simulink model "lab12"  (R2022b)
settings: Solver=VariableStepAuto  StartTime=0.0  StopTime=100  RelTol=1e-3
values from neighbouring files (symbols this model uses):
  m = 5    [lab3_1.m]    (also in lab43_2.m = 200)
  n = 7    [lab3_1.m]    (also in test.m = length(polynomial1_bin); test_OCMC.m = length(seq1))
libraries: simulink x2, dspstat3 x1
settings Model: Creator=user  LastModifiedBy=user

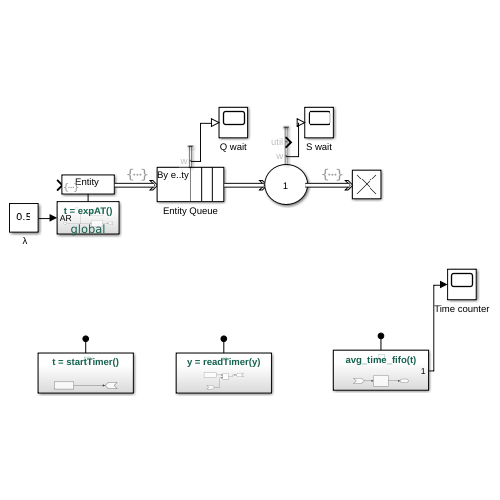
[thumbnail: Simulink's stored preview of the top-level diagram]
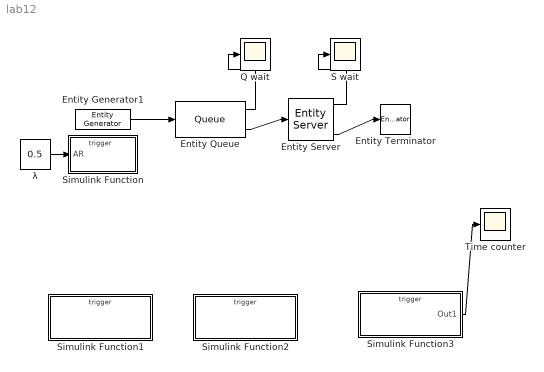
== system lab12 ==
  " λ" : Constant  Value=0.5  SampleTime=-1
  Entity Generator1 : EntityGenerator  OutputPortMessageModes=m  TimeSource=Signal port  IntergenerationTimeAction=dt = expAT();  GenerateAction=|  AttributeName=ServiceTime|Timer  AttributeInitialValue=0|0  EntityType=Structured  EntityTypeName=Entity
      | entity.ServiceTime = exprnd(3);
      | entitySys.priority = randi(2);
      | entity.Timer = 0; % Инициализация Timer
      | entity.Timer = startTimer(); % Запуск таймера
      settings: InputPortMap=u1
  Entity Queue : Queue  InputPortMessageModes=m  OutputPortMessageModes=n,m  Capacity=100  QueueType=Priority  PrioritySource=entitySys.priority  EntryAction=entity.Timer = startTimer();  AverageWait=on
      settings: OutputPortMap=o2,o5
  Entity Server : EntityServer  InputPortMessageModes=m  OutputPortMessageModes=n,n,m  Capacity=1  ServiceTimeSource=Attribute  AverageWait=on  Utilization=on
      settings: OutputPortMap=o4,o5,o9
  Entity Terminator : EntityTerminator  InputPortMessageModes=m  EntryAction=|
      | elapsedTime = readTimer(entity.Timer);
      | avg_time_fifo(elapsedTime);
  Q wait : Scope
  S wait : Scope
  Simulink Function : Subsystem  TreatAsAtomicUnit=on
      settings: LibrarySourceBlock=sldelib/Simulink Function
  Simulink Function1 : Subsystem  TreatAsAtomicUnit=on
  Simulink Function2 : Subsystem  TreatAsAtomicUnit=on
  Simulink Function3 : Subsystem  TreatAsAtomicUnit=on
  Time counter : Scope
  wires:
  " λ"/1 -> Simulink Function/1(AR)
  Entity Generator1/1 -> Entity Queue/1
  Entity Queue/2 -> Entity Server/1
  Entity Server/3 -> Entity Terminator/1
  Simulink Function3/1(Out1) -> Time counter/1
  Entity Server/1 -> S wait/1
  Entity Queue/1 -> Q wait/1

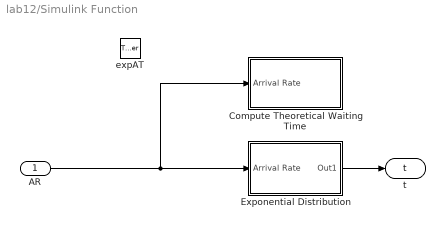
== system lab12/Simulink Function ==
  AR : Inport
  expAT : TriggerPort  TriggerType=function-call  IsSimulinkFunction=on  FunctionName=expAT  VariantControl=Variant
  Compute Theoretical Waiting Time : Subsystem
  Exponential Distribution : Subsystem
  t : ArgOut  DisableCoverage=on  ArgumentName=t
  wires:
  Exponential Distribution/1(Out1) -> t/1
  AR/1 -> Compute Theoretical Waiting Time/1(Arrival Rate), Exponential Distribution/1(Arrival Rate)

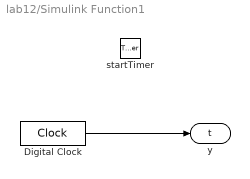
== system lab12/Simulink Function1 ==
  startTimer : TriggerPort  TriggerType=function-call  IsSimulinkFunction=on  FunctionName=startTimer  FunctionVisibility=scoped  VariantControl=(inherit)
  Digital Clock : DigitalClock  SampleTime=-1
  y : ArgOut  DisableCoverage=on  ArgumentName=t
  wires:
  Digital Clock/1 -> y/1

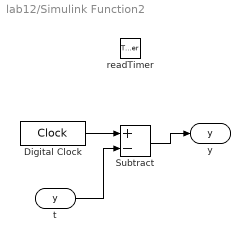
== system lab12/Simulink Function2 ==
  readTimer : TriggerPort  TriggerType=function-call  IsSimulinkFunction=on  FunctionName=readTimer  FunctionVisibility=scoped  VariantControl=(inherit)
  Digital Clock : DigitalClock  SampleTime=-1
  Subtract : Sum  Inputs=+-
  t : ArgIn  DisableCoverage=on  ArgumentName=y
  y : ArgOut  DisableCoverage=on  ArgumentName=y
  wires:
  Digital Clock/1 -> Subtract/1
  t/1 -> Subtract/2
  Subtract/1 -> y/1

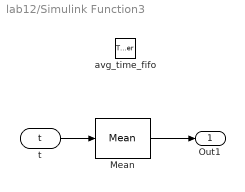
== system lab12/Simulink Function3 ==
  avg_time_fifo : TriggerPort  TriggerType=function-call  IsSimulinkFunction=on  FunctionName=avg_time_fifo  FunctionVisibility=scoped  VariantControl=(inherit)
  Mean : dspstat3/Mean  run=off  InputProcessing=Columns as channels (frame based)  reset_popup=None  directionMode=Each column  dimension=1  roiEnable=off  roiType=Rectangles  roiPortion=Entire ROI  roiOutput=Individual statistics for each ROI  roiFlag=off  roundingMode=Floor  overflowMode=off  outputDataTypeStr=Inherit: Same as accumulator  outputMin=[]  outputMax=[]  outputLastDataTypeStr=Inherit: Same as accumulator
  t : ArgIn  DisableCoverage=on  ArgumentName=t
  Out1 : Outport
  wires:
  Mean/1 -> Out1/1
  t/1 -> Mean/1

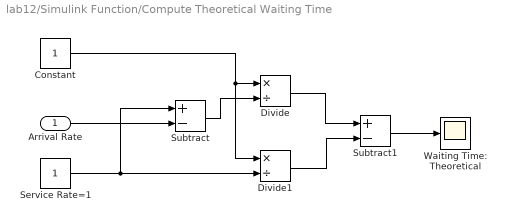
== system lab12/Simulink Function/Compute Theoretical Waiting Time ==
  Arrival Rate : Inport
  Constant : Constant
  Divide : Product  Inputs=*/
  Divide1 : Product  Inputs=*/
  Service Rate=1 : Constant
  Subtract : Sum  Inputs=+-
  Subtract1 : Sum  Inputs=+-
  Waiting Time: Theoretical : Scope
  wires:
  Arrival Rate/1 -> Subtract/2
  Subtract1/1 -> Waiting Time: Theoretical/1
  Divide1/1 -> Subtract1/2
  Divide/1 -> Subtract1/1
  Subtract/1 -> Divide/2
  Constant/1 -> Divide1/1, Divide/1
  Service Rate=1/1 -> Subtract/1, Divide1/2

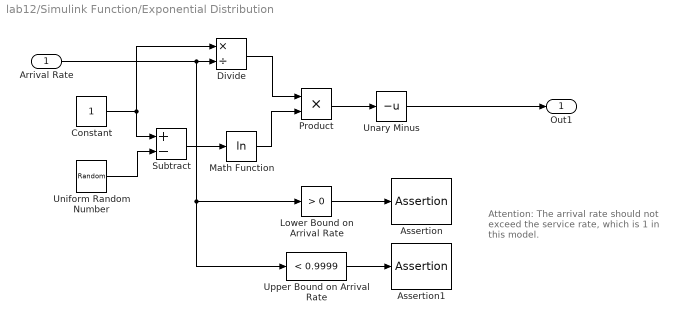
== system lab12/Simulink Function/Exponential Distribution ==
  note: Attention: The arrival rate
      | should not exceed the service
      | rate, which is 1 in this model.
  Arrival Rate : Inport
  Assertion : Assertion
  Assertion1 : Assertion
  Constant : Constant
  Divide : Product  Inputs=*/
  Lower Bound on Arrival Rate : simulink/Logic and Bit Operations/Compare To Constant  relop=>  const=0  OutDataTypeStr=uint8  ZeroCross=off
  Math Function : Math  Operator=log  SignedPower=on
  Product : Product  RndMeth=Zero
  Subtract : Sum  Inputs=+-
  Unary Minus : UnaryMinus
  Uniform Random Number : UniformRandomNumber  Minimum=0  Seed=12345
  "Upper Bound on Arrival Rate " : simulink/Logic and Bit Operations/Compare To Constant  relop=<  const=0.9999  OutDataTypeStr=uint8  ZeroCross=off
  Out1 : Outport
  wires:
  Arrival Rate/1 -> Divide/2, Lower Bound on Arrival Rate/1, "Upper Bound on Arrival Rate "/1
  Unary Minus/1 -> Out1/1
  Product/1 -> Unary Minus/1
  Math Function/1 -> Product/2
  Divide/1 -> Product/1
  Constant/1 -> Divide/1, Subtract/1
  Uniform Random Number/1 -> Subtract/2
  Lower Bound on Arrival Rate/1 -> Assertion/1
  "Upper Bound on Arrival Rate "/1 -> Assertion1/1
  Subtract/1 -> Math Function/1
